simulink model "F16A_Logical"  (R2026a)
settings: Solver=VariableStepAuto
settings Model: DataDictionary=F16A_Logical.sldd  Creator=darsh  LastModifiedBy=darsh

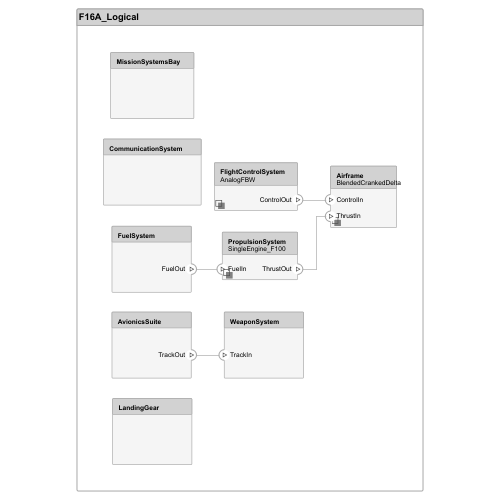
[thumbnail: Simulink's stored preview of the top-level diagram]
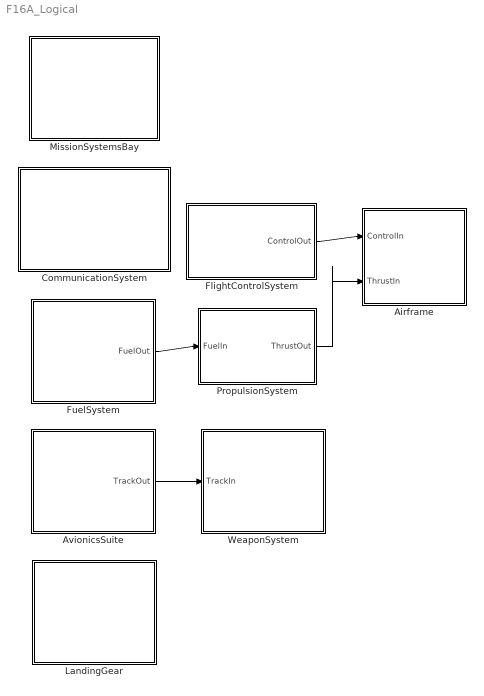
== system F16A_Logical ==
  Airframe : Subsystem  Variant=on  VariantControlMode=label  LabelModeActiveChoice=BlendedCrankedDelta
      settings: PortSchema="{\"entries\":[{\"content\":{\"headerSize\":38,\"margin\":15,\"minimumSpacing\":25,\"sides\":[{\"content\":{\"connectorIds\":[\"In1\",\"In2\"]},\"type\":\"ConnectorPlacement.EquallySpacedRectSide\",\"uuid\":\"121ec82c-bb87-4e6d-a72f-0ff4493d3409\"},{\"content\":{\"side\":\"RIGHT\"},\"type\":\"ConnectorPlacement.EquallySpacedRectSide\",\"uuid\":\"39991be8-4950-4049-85c5-6e576714a65f\"},{\"content\":{\"side\":\"TOP\"},\"type\":\"ConnectorPlacement.EquallySpacedRectSide\",\"uuid\":\"0e36527e-7320-4c10-983a-3d3da9015de0\"}]},\"type\":\"ConnectorPlacement.EquallySpacedConnector\",\"uuid\":\"ef68ad2b-b801-4b4d-b333-c00aff17ecce\"}],\"packageUris\":[\"http://schema.mathworks.com/mf0/Connector/R2020b\"],\"version\":\"1.0\"}"
  AvionicsSuite : Subsystem
      settings: PortSchema="{\"entries\":[{\"content\":{\"headerSize\":26,\"margin\":15,\"minimumSpacing\":25,\"sides\":[{\"content\":{},\"type\":\"ConnectorPlacement.EquallySpacedRectSide\",\"uuid\":\"9e7c0d22-d214-43b6-9e9e-f4b5c47205c9\"},{\"content\":{\"connectorIds\":[\"Out1\"],\"side\":\"RIGHT\"},\"type\":\"ConnectorPlacement.EquallySpacedRectSide\",\"uuid\":\"5e93f8a9-aac0-4f8f-af79-960a64193fb3\"},{\"content\":{\"side\":\"TOP\"},\"type\":\"ConnectorPlacement.EquallySpacedRectSide\",\"uuid\":\"451a3b14-5e15-45c2-b179-edf087f7dc69\"}]},\"type\":\"ConnectorPlacement.EquallySpacedConnector\",\"uuid\":\"e582b2b6-aeb3-45d4-b86c-cd2c221f80e4\"}],\"packageUris\":[\"http://schema.mathworks.com/mf0/Connector/R2020b\"],\"version\":\"1.0\"}"
  CommunicationSystem : Subsystem
      settings: PortSchema="{\"entries\":[{\"content\":{\"headerSize\":26,\"margin\":15,\"minimumSpacing\":25,\"sides\":[{\"content\":{},\"type\":\"ConnectorPlacement.EquallySpacedRectSide\",\"uuid\":\"9e7c0d22-d214-43b6-9e9e-f4b5c47205c9\"},{\"content\":{\"side\":\"RIGHT\"},\"type\":\"ConnectorPlacement.EquallySpacedRectSide\",\"uuid\":\"5e93f8a9-aac0-4f8f-af79-960a64193fb3\"},{\"content\":{\"side\":\"TOP\"},\"type\":\"ConnectorPlacement.EquallySpacedRectSide\",\"uuid\":\"451a3b14-5e15-45c2-b179-edf087f7dc69\"}]},\"type\":\"ConnectorPlacement.EquallySpacedConnector\",\"uuid\":\"e582b2b6-aeb3-45d4-b86c-cd2c221f80e4\"}],\"packageUris\":[\"http://schema.mathworks.com/mf0/Connector/R2020b\"],\"version\":\"1.0\"}"
  FlightControlSystem : Subsystem  Variant=on  VariantControlMode=label  LabelModeActiveChoice=AnalogFBW
      settings: PortSchema="{\"entries\":[{\"content\":{\"headerSize\":38,\"margin\":15,\"minimumSpacing\":25,\"sides\":[{\"content\":{},\"type\":\"ConnectorPlacement.EquallySpacedRectSide\",\"uuid\":\"121ec82c-bb87-4e6d-a72f-0ff4493d3409\"},{\"content\":{\"connectorIds\":[\"Out1\"],\"side\":\"RIGHT\"},\"type\":\"ConnectorPlacement.EquallySpacedRectSide\",\"uuid\":\"39991be8-4950-4049-85c5-6e576714a65f\"},{\"content\":{\"side\":\"TOP\"},\"type\":\"ConnectorPlacement.EquallySpacedRectSide\",\"uuid\":\"0e36527e-7320-4c10-983a-3d3da9015de0\"}]},\"type\":\"ConnectorPlacement.EquallySpacedConnector\",\"uuid\":\"ef68ad2b-b801-4b4d-b333-c00aff17ecce\"}],\"packageUris\":[\"http://schema.mathworks.com/mf0/Connector/R2020b\"],\"version\":\"1.0\"}"
  FuelSystem : Subsystem
      settings: PortSchema="{\"entries\":[{\"content\":{\"headerSize\":26,\"margin\":15,\"minimumSpacing\":25,\"sides\":[{\"content\":{},\"type\":\"ConnectorPlacement.EquallySpacedRectSide\",\"uuid\":\"9e7c0d22-d214-43b6-9e9e-f4b5c47205c9\"},{\"content\":{\"connectorIds\":[\"Out1\"],\"side\":\"RIGHT\"},\"type\":\"ConnectorPlacement.EquallySpacedRectSide\",\"uuid\":\"5e93f8a9-aac0-4f8f-af79-960a64193fb3\"},{\"content\":{\"side\":\"TOP\"},\"type\":\"ConnectorPlacement.EquallySpacedRectSide\",\"uuid\":\"451a3b14-5e15-45c2-b179-edf087f7dc69\"}]},\"type\":\"ConnectorPlacement.EquallySpacedConnector\",\"uuid\":\"e582b2b6-aeb3-45d4-b86c-cd2c221f80e4\"}],\"packageUris\":[\"http://schema.mathworks.com/mf0/Connector/R2020b\"],\"version\":\"1.0\"}"
  LandingGear : Subsystem
      settings: PortSchema="{\"entries\":[{\"content\":{\"headerSize\":26,\"margin\":15,\"minimumSpacing\":25,\"sides\":[{\"content\":{},\"type\":\"ConnectorPlacement.EquallySpacedRectSide\",\"uuid\":\"9e7c0d22-d214-43b6-9e9e-f4b5c47205c9\"},{\"content\":{\"side\":\"RIGHT\"},\"type\":\"ConnectorPlacement.EquallySpacedRectSide\",\"uuid\":\"5e93f8a9-aac0-4f8f-af79-960a64193fb3\"},{\"content\":{\"side\":\"TOP\"},\"type\":\"ConnectorPlacement.EquallySpacedRectSide\",\"uuid\":\"451a3b14-5e15-45c2-b179-edf087f7dc69\"}]},\"type\":\"ConnectorPlacement.EquallySpacedConnector\",\"uuid\":\"e582b2b6-aeb3-45d4-b86c-cd2c221f80e4\"}],\"packageUris\":[\"http://schema.mathworks.com/mf0/Connector/R2020b\"],\"version\":\"1.0\"}"
  MissionSystemsBay : Subsystem
      settings: PortSchema="{\"entries\":[{\"content\":{\"headerSize\":26,\"margin\":15,\"minimumSpacing\":25,\"sides\":[{\"content\":{},\"type\":\"ConnectorPlacement.EquallySpacedRectSide\",\"uuid\":\"9e7c0d22-d214-43b6-9e9e-f4b5c47205c9\"},{\"content\":{\"side\":\"RIGHT\"},\"type\":\"ConnectorPlacement.EquallySpacedRectSide\",\"uuid\":\"5e93f8a9-aac0-4f8f-af79-960a64193fb3\"},{\"content\":{\"side\":\"TOP\"},\"type\":\"ConnectorPlacement.EquallySpacedRectSide\",\"uuid\":\"451a3b14-5e15-45c2-b179-edf087f7dc69\"}]},\"type\":\"ConnectorPlacement.EquallySpacedConnector\",\"uuid\":\"e582b2b6-aeb3-45d4-b86c-cd2c221f80e4\"}],\"packageUris\":[\"http://schema.mathworks.com/mf0/Connector/R2020b\"],\"version\":\"1.0\"}"
  PropulsionSystem : Subsystem  Variant=on  VariantControlMode=label  LabelModeActiveChoice=SingleEngine_F100
      settings: PortSchema="{\"entries\":[{\"content\":{\"headerSize\":38,\"margin\":15,\"minimumSpacing\":25,\"sides\":[{\"content\":{\"connectorIds\":[\"In1\"]},\"type\":\"ConnectorPlacement.EquallySpacedRectSide\",\"uuid\":\"121ec82c-bb87-4e6d-a72f-0ff4493d3409\"},{\"content\":{\"connectorIds\":[\"Out1\"],\"side\":\"RIGHT\"},\"type\":\"ConnectorPlacement.EquallySpacedRectSide\",\"uuid\":\"39991be8-4950-4049-85c5-6e576714a65f\"},{\"content\":{\"side\":\"TOP\"},\"type\":\"ConnectorPlacement.EquallySpacedRectSide\",\"uuid\":\"0e36527e-7320-4c10-983a-3d3da9015de0\"}]},\"type\":\"ConnectorPlacement.EquallySpacedConnector\",\"uuid\":\"ef68ad2b-b801-4b4d-b333-c00aff17ecce\"}],\"packageUris\":[\"http://schema.mathworks.com/mf0/Connector/R2020b\"],\"version\":\"1.0\"}"
  WeaponSystem : Subsystem
      settings: PortSchema="{\"entries\":[{\"content\":{\"headerSize\":26,\"margin\":15,\"minimumSpacing\":25,\"sides\":[{\"content\":{\"connectorIds\":[\"In1\"]},\"type\":\"ConnectorPlacement.EquallySpacedRectSide\",\"uuid\":\"9e7c0d22-d214-43b6-9e9e-f4b5c47205c9\"},{\"content\":{\"side\":\"RIGHT\"},\"type\":\"ConnectorPlacement.EquallySpacedRectSide\",\"uuid\":\"5e93f8a9-aac0-4f8f-af79-960a64193fb3\"},{\"content\":{\"side\":\"TOP\"},\"type\":\"ConnectorPlacement.EquallySpacedRectSide\",\"uuid\":\"451a3b14-5e15-45c2-b179-edf087f7dc69\"}]},\"type\":\"ConnectorPlacement.EquallySpacedConnector\",\"uuid\":\"e582b2b6-aeb3-45d4-b86c-cd2c221f80e4\"}],\"packageUris\":[\"http://schema.mathworks.com/mf0/Connector/R2020b\"],\"version\":\"1.0\"}"
  wires:
  FlightControlSystem/1(ControlOut) -> Airframe/1(ControlIn)
  FuelSystem/1(FuelOut) -> PropulsionSystem/1(FuelIn)
  AvionicsSuite/1(TrackOut) -> WeaponSystem/1(TrackIn)
  PropulsionSystem/1(ThrustOut) -> Airframe/2(ThrustIn)

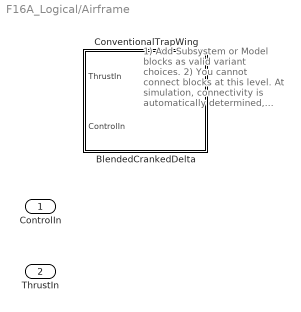
== system F16A_Logical/Airframe ==
  note: 1) Add Subsystem or Model blocks as valid variant choices.
      | 2) You cannot connect blocks at this level. At simulation, connectivity is automatically
      | determined, based on the active variant and port name matching.
  ControlIn : Inport
  ThrustIn : Inport  Port=2
  BlendedCrankedDelta : Subsystem  VariantControl=BlendedCrankedDelta
      settings: PortSchema="{\"entries\":[{\"content\":{\"headerSize\":26,\"margin\":15,\"minimumSpacing\":25,\"sides\":[{\"content\":{\"connectorIds\":[\"In1\",\"In2\"]},\"type\":\"ConnectorPlacement.EquallySpacedRectSide\",\"uuid\":\"9e7c0d22-d214-43b6-9e9e-f4b5c47205c9\"},{\"content\":{\"side\":\"RIGHT\"},\"type\":\"ConnectorPlacement.EquallySpacedRectSide\",\"uuid\":\"5e93f8a9-aac0-4f8f-af79-960a64193fb3\"},{\"content\":{\"side\":\"TOP\"},\"type\":\"ConnectorPlacement.EquallySpacedRectSide\",\"uuid\":\"451a3b14-5e15-45c2-b179-edf087f7dc69\"}]},\"type\":\"ConnectorPlacement.EquallySpacedConnector\",\"uuid\":\"e582b2b6-aeb3-45d4-b86c-cd2c221f80e4\"}],\"packageUris\":[\"http://schema.mathworks.com/mf0/Connector/R2020b\"],\"version\":\"1.0\"}"
  ConventionalTrapWing : Subsystem  VariantControl=ConventionalTrapWing
      settings: PortSchema="{\"entries\":[{\"content\":{\"headerSize\":26,\"margin\":15,\"minimumSpacing\":25,\"sides\":[{\"content\":{\"connectorIds\":[\"In1\",\"In2\"]},\"type\":\"ConnectorPlacement.EquallySpacedRectSide\",\"uuid\":\"9e7c0d22-d214-43b6-9e9e-f4b5c47205c9\"},{\"content\":{\"side\":\"RIGHT\"},\"type\":\"ConnectorPlacement.EquallySpacedRectSide\",\"uuid\":\"5e93f8a9-aac0-4f8f-af79-960a64193fb3\"},{\"content\":{\"side\":\"TOP\"},\"type\":\"ConnectorPlacement.EquallySpacedRectSide\",\"uuid\":\"451a3b14-5e15-45c2-b179-edf087f7dc69\"}]},\"type\":\"ConnectorPlacement.EquallySpacedConnector\",\"uuid\":\"e582b2b6-aeb3-45d4-b86c-cd2c221f80e4\"}],\"packageUris\":[\"http://schema.mathworks.com/mf0/Connector/R2020b\"],\"version\":\"1.0\"}"

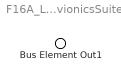
== system F16A_Logical/AvionicsSuite ==
  Bus Element Out1 : Outport  PortName=TrackOut

== system F16A_Logical/CommunicationSystem ==

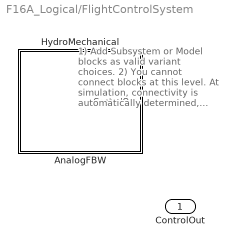
== system F16A_Logical/FlightControlSystem ==
  note: 1) Add Subsystem or Model blocks as valid variant choices.
      | 2) You cannot connect blocks at this level. At simulation, connectivity is automatically
      | determined, based on the active variant and port name matching.
  AnalogFBW : Subsystem  VariantControl=AnalogFBW
      settings: PortSchema="{\"entries\":[{\"content\":{\"headerSize\":26,\"margin\":15,\"minimumSpacing\":25,\"sides\":[{\"content\":{},\"type\":\"ConnectorPlacement.EquallySpacedRectSide\",\"uuid\":\"9e7c0d22-d214-43b6-9e9e-f4b5c47205c9\"},{\"content\":{\"connectorIds\":[\"Out1\"],\"side\":\"RIGHT\"},\"type\":\"ConnectorPlacement.EquallySpacedRectSide\",\"uuid\":\"5e93f8a9-aac0-4f8f-af79-960a64193fb3\"},{\"content\":{\"side\":\"TOP\"},\"type\":\"ConnectorPlacement.EquallySpacedRectSide\",\"uuid\":\"451a3b14-5e15-45c2-b179-edf087f7dc69\"}]},\"type\":\"ConnectorPlacement.EquallySpacedConnector\",\"uuid\":\"e582b2b6-aeb3-45d4-b86c-cd2c221f80e4\"}],\"packageUris\":[\"http://schema.mathworks.com/mf0/Connector/R2020b\"],\"version\":\"1.0\"}"
  HydroMechanical : Subsystem  VariantControl=HydroMechanical
      settings: PortSchema="{\"entries\":[{\"content\":{\"headerSize\":26,\"margin\":15,\"minimumSpacing\":25,\"sides\":[{\"content\":{},\"type\":\"ConnectorPlacement.EquallySpacedRectSide\",\"uuid\":\"9e7c0d22-d214-43b6-9e9e-f4b5c47205c9\"},{\"content\":{\"connectorIds\":[\"Out1\"],\"side\":\"RIGHT\"},\"type\":\"ConnectorPlacement.EquallySpacedRectSide\",\"uuid\":\"5e93f8a9-aac0-4f8f-af79-960a64193fb3\"},{\"content\":{\"side\":\"TOP\"},\"type\":\"ConnectorPlacement.EquallySpacedRectSide\",\"uuid\":\"451a3b14-5e15-45c2-b179-edf087f7dc69\"}]},\"type\":\"ConnectorPlacement.EquallySpacedConnector\",\"uuid\":\"e582b2b6-aeb3-45d4-b86c-cd2c221f80e4\"}],\"packageUris\":[\"http://schema.mathworks.com/mf0/Connector/R2020b\"],\"version\":\"1.0\"}"
  ControlOut : Outport

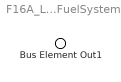
== system F16A_Logical/FuelSystem ==
  Bus Element Out1 : Outport  PortName=FuelOut

== system F16A_Logical/LandingGear ==

== system F16A_Logical/MissionSystemsBay ==

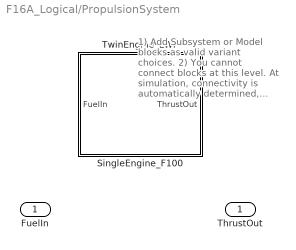
== system F16A_Logical/PropulsionSystem ==
  note: 1) Add Subsystem or Model blocks as valid variant choices.
      | 2) You cannot connect blocks at this level. At simulation, connectivity is automatically
      | determined, based on the active variant and port name matching.
  FuelIn : Inport
  SingleEngine_F100 : Subsystem  VariantControl=SingleEngine_F100
      settings: PortSchema="{\"entries\":[{\"content\":{\"headerSize\":26,\"margin\":15,\"minimumSpacing\":25,\"sides\":[{\"content\":{\"connectorIds\":[\"In1\"]},\"type\":\"ConnectorPlacement.EquallySpacedRectSide\",\"uuid\":\"9e7c0d22-d214-43b6-9e9e-f4b5c47205c9\"},{\"content\":{\"connectorIds\":[\"Out1\"],\"side\":\"RIGHT\"},\"type\":\"ConnectorPlacement.EquallySpacedRectSide\",\"uuid\":\"5e93f8a9-aac0-4f8f-af79-960a64193fb3\"},{\"content\":{\"side\":\"TOP\"},\"type\":\"ConnectorPlacement.EquallySpacedRectSide\",\"uuid\":\"451a3b14-5e15-45c2-b179-edf087f7dc69\"}]},\"type\":\"ConnectorPlacement.EquallySpacedConnector\",\"uuid\":\"e582b2b6-aeb3-45d4-b86c-cd2c221f80e4\"}],\"packageUris\":[\"http://schema.mathworks.com/mf0/Connector/R2020b\"],\"version\":\"1.0\"}"
  TwinEngine_LWF : Subsystem  VariantControl=TwinEngine_LWF
      settings: PortSchema="{\"entries\":[{\"content\":{\"headerSize\":26,\"margin\":15,\"minimumSpacing\":25,\"sides\":[{\"content\":{\"connectorIds\":[\"In1\"]},\"type\":\"ConnectorPlacement.EquallySpacedRectSide\",\"uuid\":\"9e7c0d22-d214-43b6-9e9e-f4b5c47205c9\"},{\"content\":{\"connectorIds\":[\"Out1\"],\"side\":\"RIGHT\"},\"type\":\"ConnectorPlacement.EquallySpacedRectSide\",\"uuid\":\"5e93f8a9-aac0-4f8f-af79-960a64193fb3\"},{\"content\":{\"side\":\"TOP\"},\"type\":\"ConnectorPlacement.EquallySpacedRectSide\",\"uuid\":\"451a3b14-5e15-45c2-b179-edf087f7dc69\"}]},\"type\":\"ConnectorPlacement.EquallySpacedConnector\",\"uuid\":\"e582b2b6-aeb3-45d4-b86c-cd2c221f80e4\"}],\"packageUris\":[\"http://schema.mathworks.com/mf0/Connector/R2020b\"],\"version\":\"1.0\"}"
  ThrustOut : Outport

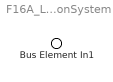
== system F16A_Logical/WeaponSystem ==
  Bus Element In1 : Inport  PortName=TrackIn

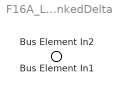
== system F16A_Logical/Airframe/BlendedCrankedDelta ==
  Bus Element In1 : Inport  PortName=ThrustIn
  Bus Element In2 : Inport  Port=2  PortName=ControlIn

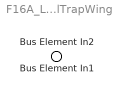
== system F16A_Logical/Airframe/ConventionalTrapWing ==
  Bus Element In1 : Inport  PortName=ThrustIn
  Bus Element In2 : Inport  Port=2  PortName=ControlIn

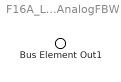
== system F16A_Logical/FlightControlSystem/AnalogFBW ==
  Bus Element Out1 : Outport  PortName=ControlOut

== system F16A_Logical/FlightControlSystem/HydroMechanical ==
  Bus Element Out1 : Outport  PortName=ControlOut

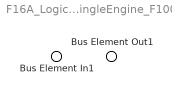
== system F16A_Logical/PropulsionSystem/SingleEngine_F100 ==
  Bus Element In1 : Inport  PortName=FuelIn
  Bus Element Out1 : Outport  PortName=ThrustOut

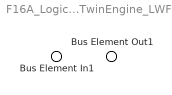
== system F16A_Logical/PropulsionSystem/TwinEngine_LWF ==
  Bus Element In1 : Inport  PortName=FuelIn
  Bus Element Out1 : Outport  PortName=ThrustOut
